simulink model "Modelo5_1_2_C_4"  (R2020a)
settings: Solver=VariableStepAuto  StartTime=0.0  StopTime=10.0  RelTol=1e-3
values from neighbouring files (symbols this model uses):
  Cts = 0.818    [AnalisisDeEstabilidad.m]
  Ld = 5.8e-3    (= 0.0058)    [AnalisisDeEstabilidad.m]
  Lls = 0.8e-3    (= 0.0008)    [AnalisisDeEstabilidad.m]
  Lq = 6.6e-3    (= 0.0066)    [AnalisisDeEstabilidad.m]
  Pp = 3    [AnalisisDeEstabilidad.m]    (also in LTI_vs_LPV_vs_NL_realimentado.m; Modelo_linealizado.m; parametros.m)
  r = 120    [AnalisisDeEstabilidad.m]    (also in LTI_vs_LPV_vs_NL_realimentado.m; Modelo_linealizado.m; parametros.m)
  Rsref = 1.02    [AnalisisDeEstabilidad.m]
  Rts = 146.7    [AnalisisDeEstabilidad.m]
  Tref = 25    [AnalisisDeEstabilidad.m]
undefined symbols (not defined in the file or in its folder): aa, beq, Jeq, Kl, lam
settings Model: Creator=matie  LastModifiedBy=matie

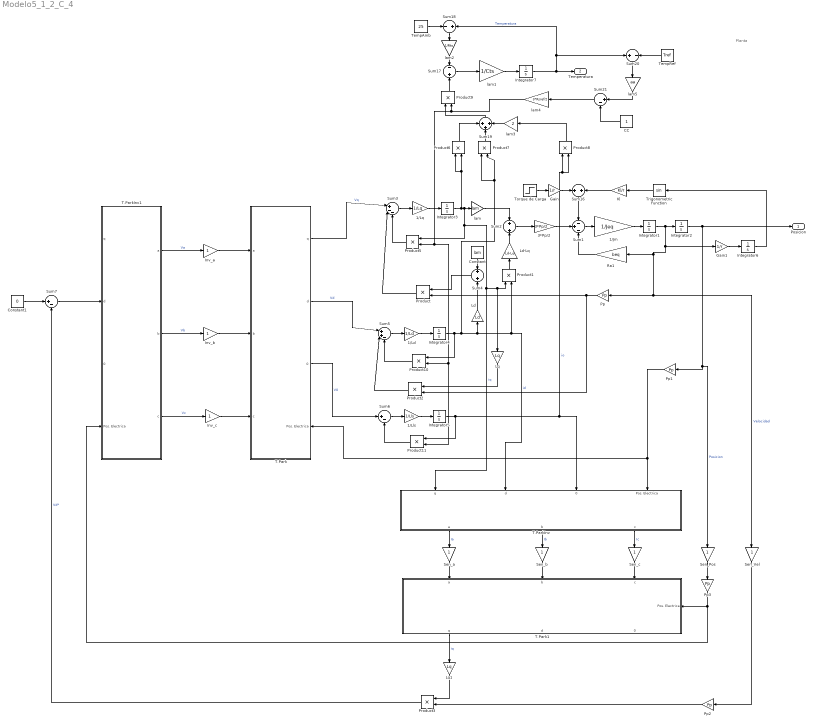
== system Modelo5_1_2_C_4 ==
  note: Planta
  1/Jm : Gain  Gain=1/Jeq
  1/Ld : Gain  Gain=1/Ld
  1/Lls : Gain  Gain=1/Lls
  1/Lq : Gain  Gain=1/Lq
  3*Pp/2 : Gain  Gain=3*Pp/2
  CC : Constant
  Constant : Constant  Value=lam
  Constant1 : Constant  Value=0
  Gain : Gain  Gain=1/r
  Gain1 : Gain  Gain=1/r
  Integrator{1..7} (7 alike) : Integrator
  Inv_a : Gain
  Inv_b : Gain
  Inv_c : Gain
  Kl : Gain  Gain=Kl/r
  Ld : Gain  Gain=Ld
  Ld-Lq : Gain  Gain=Ld-Lq
  Lq : Gain  Gain=Lq
  Lq1 : Gain  Gain=Lq
  Pp{,1..3} (4 alike) : Gain  Gain=Pp
  Product{,1..3,5..11} (11 alike) : Product
  Ra1 : Gain  Gain=beq
  Sen_Pos : Gain
  Sen_Vel : Gain
  Sen_a : Gain
  Sen_b : Gain
  Sen_c : Gain
  Sum1 : Sum  Inputs=-+-
  Sum16 : Sum  Inputs=+|+
  Sum17 : Sum  Inputs=-+
  Sum18 : Sum  Inputs=-+
  Sum19 : Sum  Inputs=+++
  Sum2 : Sum
  Sum20 : Sum  Inputs=+-
  Sum21 : Sum  Inputs=|+-
  Sum3 : Sum  Inputs=|+--
  Sum4 : Sum
  Sum5 : Sum  Inputs=|++-
  Sum6 : Sum  Inputs=|+-
  Sum7 : Sum  Inputs=|+-
  T.Park : Subsystem
      settings: PortSchema="{\"entries\":[{\"content\":{\"sides\":[{\"content\":{\"connectorIds\":[\"In1\",\"In2\",\"In3\"]},\"type\":\"ConnectorPlacement.EquallySpacedRectSide\",\"uuid\":\"2bfbe7ef-652a-4797-b13c-b84c243bd68c\"},{\"content\":{\"connectorIds\":[\"Out1\",\"Out2\",\"Out3\",\"In4\"],\"side\":\"RIGHT\"},\"type\":\"ConnectorPlacement.EquallySpacedRectSide\",\"uuid\":\"075def0e-c436-44dc-ba25-82cf6ffae869\"},{\"content\":{\"connectorIds\":[],\"side\":\"TOP\"},\"type\":\"ConnectorPlacement.EquallySpacedRectSide\",\"uuid\":\"95d81334-e332-4f04-a2cb-c4692f91809c\"}]},\"type\":\"ConnectorPlacement.EquallySpacedConnector\",\"uuid\":\"b90f9cad-0277-459c-bcac-17172872a787\"}],\"packageUris\":[\"http://schema.mathworks.com/mf0/Connector/19700101\"],\"version\":\"1.0\"}"
  T.Park1 : Subsystem
      settings: PortSchema="{\"entries\":[{\"content\":{\"sides\":[{\"content\":{\"connectorIds\":[\"In1\",\"In2\",\"In3\"]},\"type\":\"ConnectorPlacement.EquallySpacedRectSide\",\"uuid\":\"2bfbe7ef-652a-4797-b13c-b84c243bd68c\"},{\"content\":{\"connectorIds\":[\"Out1\",\"Out2\",\"Out3\"],\"side\":\"RIGHT\"},\"type\":\"ConnectorPlacement.EquallySpacedRectSide\",\"uuid\":\"075def0e-c436-44dc-ba25-82cf6ffae869\"},{\"content\":{\"connectorIds\":[],\"side\":\"TOP\"},\"type\":\"ConnectorPlacement.EquallySpacedRectSide\",\"uuid\":\"95d81334-e332-4f04-a2cb-c4692f91809c\"},{\"content\":{\"connectorIds\":[\"In4\"],\"side\":\"BOTTOM\"},\"type\":\"ConnectorPlacement.EquallySpacedRectSide\",\"uuid\":\"85b95360-e43d-49d1-a18f-690334b045e6\"}]},\"type\":\"ConnectorPlacement.EquallySpacedConnector\",\"uuid\":\"b90f9cad-0277-459c-bcac-17172872a787\"}],\"packageUris\":[\"http://schema.mathworks.com/mf0/Connector/19700101\"],\"version\":\"1.0\"}"
  T.ParkInv : Subsystem
  T.ParkInv1 : Subsystem
  TempAmb : Constant  Value=25
  TempRef : Constant  Value=Tref
  Torque de Carga : Step  Time=3  After=0  SampleTime=0
  Trigonometric Function : Trigonometry
  lam : Gain  Gain=lam
  lam1 : Gain  Gain=1/Cts
  lam2 : Gain  Gain=1/Rts
  lam3 : Gain  Gain=2
  lam4 : Gain  Gain=3*Rsref/2
  lam5 : Gain  Gain=aa
  Posicion : Outport
  Temperatura : Outport  Port=2
  wires:
  CC/1 -> Sum21/2
  Integrator7/1 -> Sum18/2, Sum20/1, Temperatura/1  "Temperatura"
  Kl/1 -> Sum16/2
  Torque de Carga/1 -> Gain/1
  lam3/1 -> Sum19/3
  TempAmb/1 -> Sum18/1
  Sum18/1 -> lam2/1
  Product6/1 -> Sum19/1
  lam2/1 -> Sum17/1
  Trigonometric Function/1 -> Kl/1
  lam1/1 -> Integrator7/1
  T.ParkInv1/3(c) -> Inv_c/1  "Vc"
  Integrator6/1 -> Trigonometric Function/1
  Gain1/1 -> Integrator6/1
  Sum17/1 -> lam1/1
  1/Lls/1 -> Integrator5/1
  Sum5/1 -> 1/Ld/1
  lam/1 -> Sum2/1
  Ld/1 -> Sum4/2
  T.ParkInv1/2(b) -> Inv_b/1  "Vb"
  Lq1/1 -> Product3/1
  Sum16/1 -> Sum1/1
  1/Ld/1 -> Integrator4/1
  Ld-Lq/1 -> Sum2/2
  T.ParkInv1/1(a) -> Inv_a/1  "Va"
  Integrator4/1 -> Product10/1, Product7/1, Product7/2, Product1/2, T.ParkInv/2(d), Ld/1  "id"
  Sum4/1 -> Product/1
  T.Park1/1(q) -> Lq1/1  "iq"
  Pp2/1 -> Product3/2
  Pp/1 -> Product2/2, Product/2
  T.ParkInv/3(c) -> Sen_c/1  "Ic"
  Pp1/1 -> T.Park/4(Pos. Electrica), T.ParkInv/4(Pos. Electrica)
  T.ParkInv/2(b) -> Sen_b/1  "Ib"
  Product/1 -> Sum3/2
  Product10/1 -> Sum5/3
  T.Park/3(0) -> Sum6/1  "V0"
  Sum6/1 -> 1/Lls/1
  Product11/1 -> Sum6/2
  Integrator2/1 -> Sen_Pos/1, Pp1/1, Posicion/1  "Posicion"
  Product1/1 -> Ld-Lq/1
  T.Park/2(d) -> Sum5/1  "Vd"
  T.Park/1(q) -> Sum3/1  "Vq"
  Sum3/1 -> 1/Lq/1
  3*Pp/2/1 -> Sum1/2
  Sum2/1 -> 3*Pp/2/1
  Lq/1 -> Product2/1
  Ra1/1 -> Sum1/3
  Constant/1 -> Sum4/1
  Product2/1 -> Sum5/2
  Sum21/1 -> lam4/1
  Product7/1 -> Sum19/2
  Integrator5/1 -> Product11/1, T.ParkInv/3(0), Product8/2, Product8/1  "io"
  Integrator1/1 -> Gain1/1, Sen_Vel/1, Pp/1, Ra1/1, Integrator2/1  "Velocidad"
  Product5/1 -> Sum3/3
  Product8/1 -> lam3/1
  Integrator3/1 -> Product6/1, Product6/2, Product5/1, Product1/1, Lq/1, T.ParkInv/1(q), lam/1  "iq"
  lam5/1 -> Sum21/1
  1/Lq/1 -> Integrator3/1
  1/Jm/1 -> Integrator1/1
  Sum20/1 -> lam5/1
  Gain/1 -> Sum16/1
  TempRef/1 -> Sum20/2
  T.ParkInv/1(a) -> Sen_a/1  "Ia"
  Product9/1 -> Sum17/2
  lam4/1 -> Product11/2, Product10/2, Product5/2, Product9/2
  Sum19/1 -> Product9/1
  Sum1/1 -> 1/Jm/1
  Inv_a/1 -> T.Park/1(a)
  Inv_b/1 -> T.Park/2(b)
  Inv_c/1 -> T.Park/3(c)
  Sen_a/1 -> T.Park1/1(a)
  Sen_b/1 -> T.Park1/2(b)
  Sen_c/1 -> T.Park1/3(c)
  Sen_Pos/1 -> Pp3/1
  Pp3/1 -> T.ParkInv1/4(Pos. Electrica), T.Park1/4(Pos. Electrica)
  Sum7/1 -> T.ParkInv1/2(d)
  Constant1/1 -> Sum7/1
  Product3/1 -> Sum7/2  "Vd*"
  Sen_Vel/1 -> Pp2/1

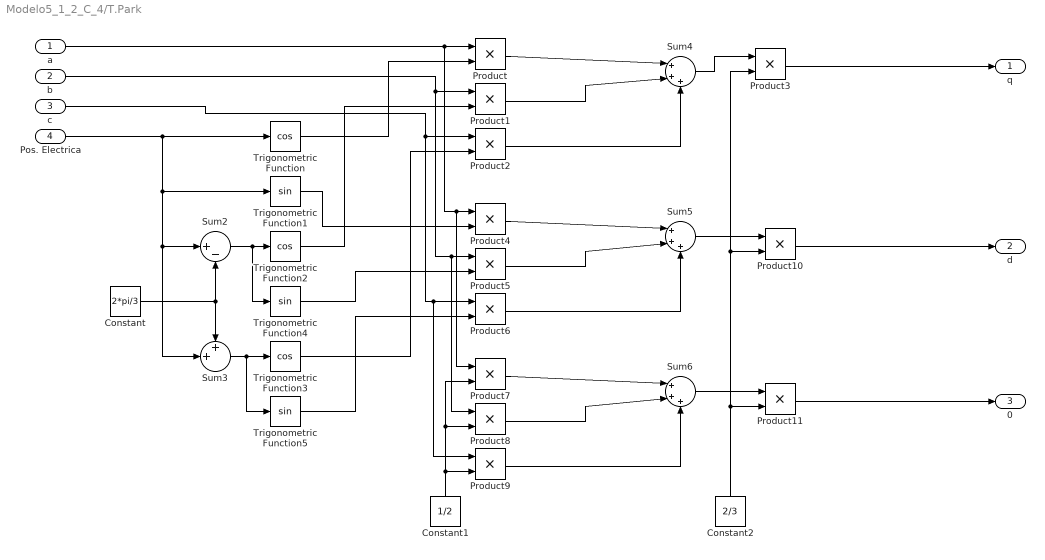
== system Modelo5_1_2_C_4/T.Park ==
  a : Inport
  b : Inport  Port=2
  c : Inport  Port=3
  Pos. Electrica : Inport  Port=4
  Constant : Constant  Value=2*pi/3
  Constant1 : Constant  Value=1/2
  Constant2 : Constant  Value=2/3
  Product{,1..11} (12 alike) : Product
  Sum2 : Sum  Inputs=|+-
  Sum3 : Sum  Inputs=++|
  Sum4 : Sum  Inputs=|+++
  Sum5 : Sum  Inputs=|+++
  Sum6 : Sum  Inputs=|+++
  Trigonometric Function : Trigonometry  Operator=cos
  Trigonometric Function1 : Trigonometry
  Trigonometric Function2 : Trigonometry  Operator=cos
  Trigonometric Function3 : Trigonometry  Operator=cos
  Trigonometric Function4 : Trigonometry
  Trigonometric Function5 : Trigonometry
  q : Outport
  d : Outport  Port=2
  0 : Outport  Port=3
  wires:
  Product1/1 -> Sum4/2
  c/1 -> Product9/1, Product6/1, Product2/1
  Constant1/1 -> Product9/2, Product8/2, Product7/2
  Sum2/1 -> Trigonometric Function4/1, Trigonometric Function2/1
  Constant2/1 -> Product11/2, Product10/2, Product3/2
  b/1 -> Product8/1, Product5/1, Product1/1
  Product11/1 -> 0/1
  Pos. Electrica/1 -> Sum3/2, Sum2/1, Trigonometric Function1/1, Trigonometric Function/1
  Trigonometric Function2/1 -> Product1/2
  Trigonometric Function5/1 -> Product6/2
  Product6/1 -> Sum5/3
  Trigonometric Function1/1 -> Product4/2
  Constant/1 -> Sum3/1, Sum2/2
  Sum5/1 -> Product10/1
  Product3/1 -> q/1
  Sum4/1 -> Product3/1
  Trigonometric Function3/1 -> Product2/2
  Trigonometric Function/1 -> Product/2
  a/1 -> Product7/1, Product4/1, Product/1
  Product10/1 -> d/1
  Trigonometric Function4/1 -> Product5/2
  Product/1 -> Sum4/1
  Product7/1 -> Sum6/1
  Sum3/1 -> Trigonometric Function5/1, Trigonometric Function3/1
  Product2/1 -> Sum4/3
  Product9/1 -> Sum6/3
  Product5/1 -> Sum5/2
  Product4/1 -> Sum5/1
  Sum6/1 -> Product11/1
  Product8/1 -> Sum6/2

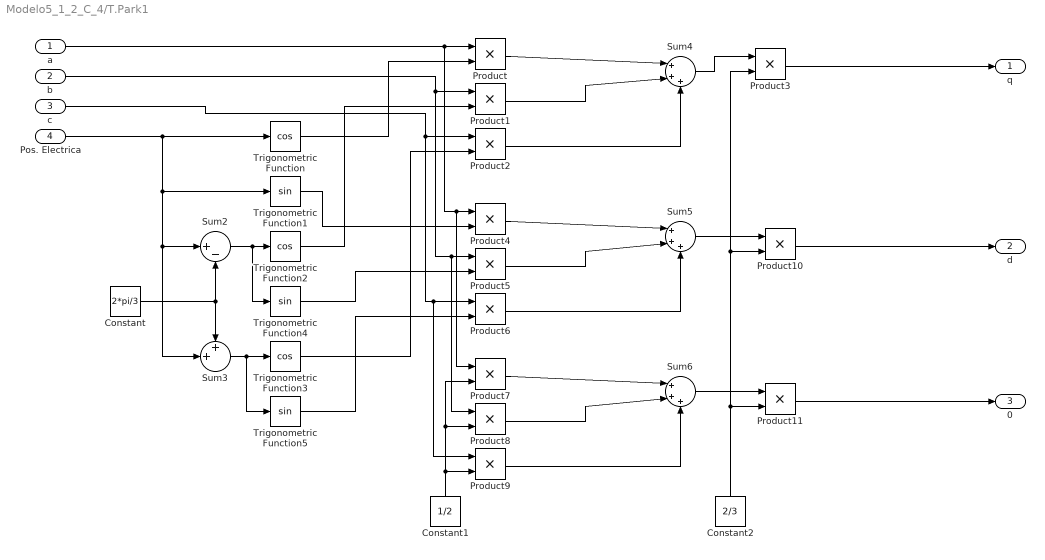
== system Modelo5_1_2_C_4/T.Park1 ==
  a : Inport
  b : Inport  Port=2
  c : Inport  Port=3
  Pos. Electrica : Inport  Port=4
  Constant : Constant  Value=2*pi/3
  Constant1 : Constant  Value=1/2
  Constant2 : Constant  Value=2/3
  Product{,1..11} (12 alike) : Product
  Sum2 : Sum  Inputs=|+-
  Sum3 : Sum  Inputs=++|
  Sum4 : Sum  Inputs=|+++
  Sum5 : Sum  Inputs=|+++
  Sum6 : Sum  Inputs=|+++
  Trigonometric Function : Trigonometry  Operator=cos
  Trigonometric Function1 : Trigonometry
  Trigonometric Function2 : Trigonometry  Operator=cos
  Trigonometric Function3 : Trigonometry  Operator=cos
  Trigonometric Function4 : Trigonometry
  Trigonometric Function5 : Trigonometry
  q : Outport
  d : Outport  Port=2
  0 : Outport  Port=3
  wires:
  Product1/1 -> Sum4/2
  c/1 -> Product9/1, Product6/1, Product2/1
  Constant1/1 -> Product9/2, Product8/2, Product7/2
  Sum2/1 -> Trigonometric Function4/1, Trigonometric Function2/1
  Constant2/1 -> Product11/2, Product10/2, Product3/2
  b/1 -> Product8/1, Product5/1, Product1/1
  Product11/1 -> 0/1
  Pos. Electrica/1 -> Sum3/2, Sum2/1, Trigonometric Function1/1, Trigonometric Function/1
  Trigonometric Function2/1 -> Product1/2
  Trigonometric Function5/1 -> Product6/2
  Product6/1 -> Sum5/3
  Trigonometric Function1/1 -> Product4/2
  Constant/1 -> Sum3/1, Sum2/2
  Sum5/1 -> Product10/1
  Product3/1 -> q/1
  Sum4/1 -> Product3/1
  Trigonometric Function3/1 -> Product2/2
  Trigonometric Function/1 -> Product/2
  a/1 -> Product7/1, Product4/1, Product/1
  Product10/1 -> d/1
  Trigonometric Function4/1 -> Product5/2
  Product/1 -> Sum4/1
  Product7/1 -> Sum6/1
  Sum3/1 -> Trigonometric Function5/1, Trigonometric Function3/1
  Product2/1 -> Sum4/3
  Product9/1 -> Sum6/3
  Product5/1 -> Sum5/2
  Product4/1 -> Sum5/1
  Sum6/1 -> Product11/1
  Product8/1 -> Sum6/2

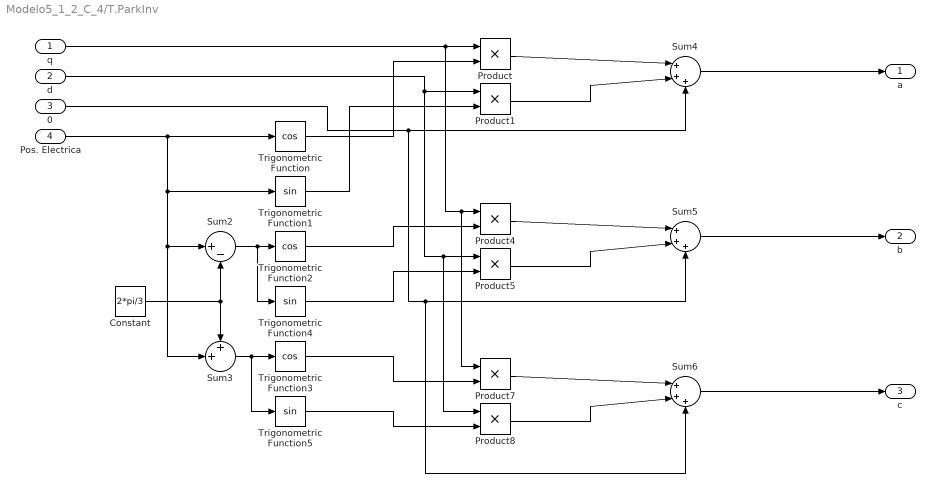
== system Modelo5_1_2_C_4/T.ParkInv ==
  q : Inport
  d : Inport  Port=2
  0 : Inport  Port=3
  Pos. Electrica : Inport  Port=4
  Constant : Constant  Value=2*pi/3
  Product{,1,4..5,7..8} (6 alike) : Product
  Sum2 : Sum  Inputs=|+-
  Sum3 : Sum  Inputs=++|
  Sum4 : Sum  Inputs=|+++
  Sum5 : Sum  Inputs=|+++
  Sum6 : Sum  Inputs=|+++
  Trigonometric Function : Trigonometry  Operator=cos
  Trigonometric Function1 : Trigonometry
  Trigonometric Function2 : Trigonometry  Operator=cos
  Trigonometric Function3 : Trigonometry  Operator=cos
  Trigonometric Function4 : Trigonometry
  Trigonometric Function5 : Trigonometry
  a : Outport
  b : Outport  Port=2
  c : Outport  Port=3
  wires:
  Constant/1 -> Sum3/1, Sum2/2
  Pos. Electrica/1 -> Sum3/2, Sum2/1, Trigonometric Function1/1, Trigonometric Function/1
  Trigonometric Function3/1 -> Product7/2
  d/1 -> Product8/1, Product5/1, Product1/1
  0/1 -> Sum4/3, Sum5/3, Sum6/3
  Product8/1 -> Sum6/2
  Product7/1 -> Sum6/1
  q/1 -> Product7/1, Product4/1, Product/1
  Sum3/1 -> Trigonometric Function5/1, Trigonometric Function3/1
  Trigonometric Function5/1 -> Product8/2
  Sum6/1 -> c/1
  Product1/1 -> Sum4/2
  Sum2/1 -> Trigonometric Function4/1, Trigonometric Function2/1
  Sum4/1 -> a/1
  Sum5/1 -> b/1
  Trigonometric Function1/1 -> Product1/2
  Product5/1 -> Sum5/2
  Trigonometric Function2/1 -> Product4/2
  Product4/1 -> Sum5/1
  Product/1 -> Sum4/1
  Trigonometric Function/1 -> Product/2
  Trigonometric Function4/1 -> Product5/2

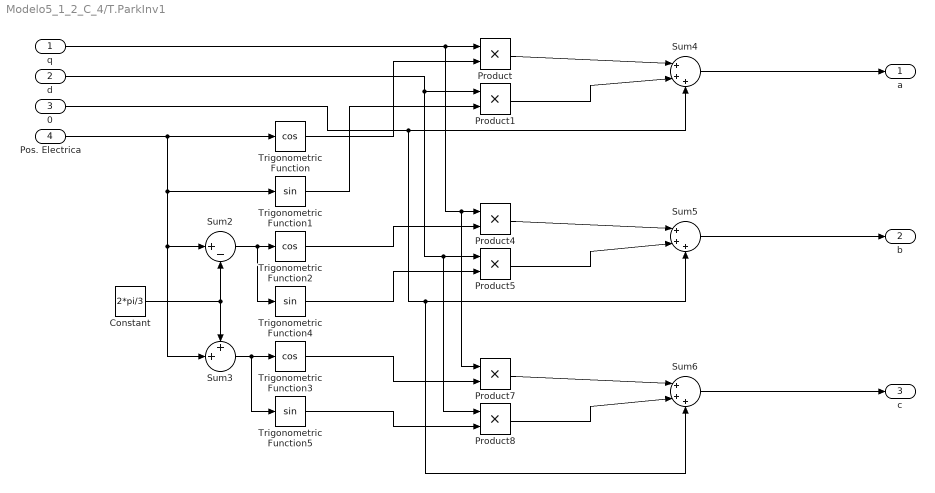
== system Modelo5_1_2_C_4/T.ParkInv1 ==
  q : Inport
  d : Inport  Port=2
  0 : Inport  Port=3
  Pos. Electrica : Inport  Port=4
  Constant : Constant  Value=2*pi/3
  Product{,1,4..5,7..8} (6 alike) : Product
  Sum2 : Sum  Inputs=|+-
  Sum3 : Sum  Inputs=++|
  Sum4 : Sum  Inputs=|+++
  Sum5 : Sum  Inputs=|+++
  Sum6 : Sum  Inputs=|+++
  Trigonometric Function : Trigonometry  Operator=cos
  Trigonometric Function1 : Trigonometry
  Trigonometric Function2 : Trigonometry  Operator=cos
  Trigonometric Function3 : Trigonometry  Operator=cos
  Trigonometric Function4 : Trigonometry
  Trigonometric Function5 : Trigonometry
  a : Outport
  b : Outport  Port=2
  c : Outport  Port=3
  wires:
  Constant/1 -> Sum3/1, Sum2/2
  Pos. Electrica/1 -> Sum3/2, Sum2/1, Trigonometric Function1/1, Trigonometric Function/1
  Trigonometric Function3/1 -> Product7/2
  d/1 -> Product8/1, Product5/1, Product1/1
  0/1 -> Sum4/3, Sum5/3, Sum6/3
  Product8/1 -> Sum6/2
  Product7/1 -> Sum6/1
  q/1 -> Product7/1, Product4/1, Product/1
  Sum3/1 -> Trigonometric Function5/1, Trigonometric Function3/1
  Trigonometric Function5/1 -> Product8/2
  Sum6/1 -> c/1
  Product1/1 -> Sum4/2
  Sum2/1 -> Trigonometric Function4/1, Trigonometric Function2/1
  Sum4/1 -> a/1
  Sum5/1 -> b/1
  Trigonometric Function1/1 -> Product1/2
  Product5/1 -> Sum5/2
  Trigonometric Function2/1 -> Product4/2
  Product4/1 -> Sum5/1
  Product/1 -> Sum4/1
  Trigonometric Function/1 -> Product/2
  Trigonometric Function4/1 -> Product5/2
